simulink library "OFDM_Rx"  (R2020a)
settings: Solver=VariableStepAuto  StartTime=0.0  StopTime=10.0  RelTol=1e-3
undefined symbols (not defined in the file): fs, LTSfreq, pilot, read_addr_rx, sc_index
libraries: simulink x36, hdlsllib x24, dsphdlmathfun x3, dsphdlxfrm x1, dsphdlsigops x1
(part 2 of 3)

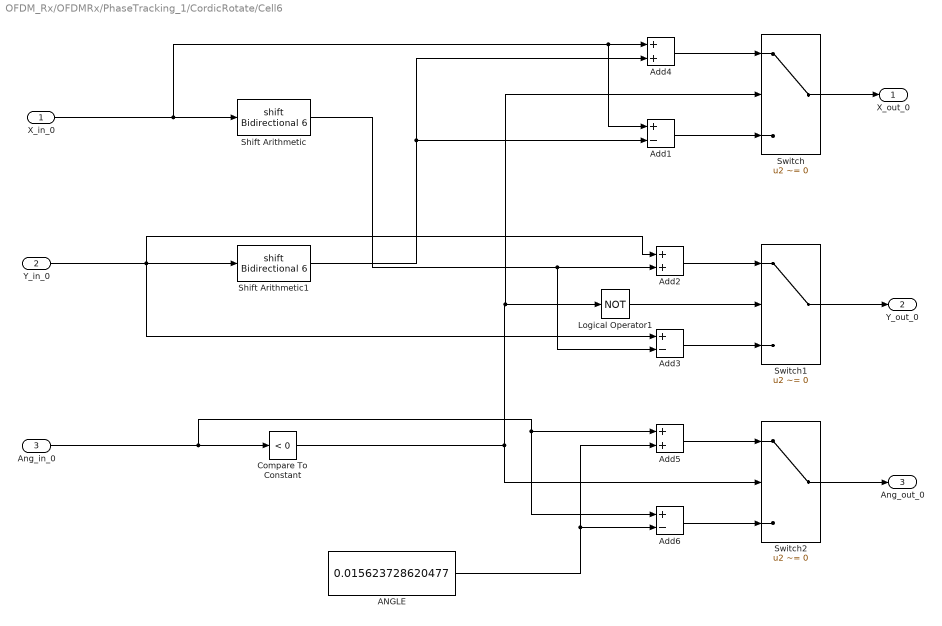
== system OFDM_Rx/OFDMRx/PhaseTracking_1/CordicRotate/Cell6 ==
  X_in_0 : Inport
  Y_in_0 : Inport  Port=2
  Ang_in_0 : Inport  Port=3
  ANGLE : Constant  Value=0.015623728620477  VectorParams1D=off  OutDataTypeStr=fixdt(1,23,20)  SampleTime=1/fs
  Add1 : Sum  Inputs=+-  OutDataTypeStr=fixdt(1,21,15)
  Add2 : Sum  OutDataTypeStr=fixdt(1,21,15)
  Add3 : Sum  Inputs=+-  OutDataTypeStr=fixdt(1,21,15)
  Add4 : Sum  OutDataTypeStr=fixdt(1,21,15)
  Add5 : Sum  OutDataTypeStr=fixdt(1,23,20)
  Add6 : Sum  Inputs=+-  OutDataTypeStr=fixdt(1,23,20)
  Compare To Constant : simulink/Logic and Bit Operations/Compare To Constant  relop=<  const=0  OutDataTypeStr=boolean
  Logical Operator1 : Logic  Operator=NOT  IconShape=distinctive  AllPortsSameDT=off  OutDataTypeStr=boolean
  Shift Arithmetic : ArithShift  BitShiftNumber=6
  Shift Arithmetic1 : ArithShift  BitShiftNumber=6
  Switch : Switch  Criteria=u2 ~= 0
  Switch1 : Switch  Criteria=u2 ~= 0
  Switch2 : Switch  Criteria=u2 ~= 0
  X_out_0 : Outport  VectorParamsAs1DForOutWhenUnconnected=off
  Y_out_0 : Outport  Port=2  VectorParamsAs1DForOutWhenUnconnected=off
  Ang_out_0 : Outport  Port=3  VectorParamsAs1DForOutWhenUnconnected=off
  wires:
  Add4/1 -> Switch/1
  Add1/1 -> Switch/3
  Add3/1 -> Switch1/3
  Add2/1 -> Switch1/1
  Switch/1 -> X_out_0/1
  Switch1/1 -> Y_out_0/1
  Add6/1 -> Switch2/3
  Add5/1 -> Switch2/1
  Switch2/1 -> Ang_out_0/1
  X_in_0/1 -> Shift Arithmetic/1, Add1/1, Add4/1
  Y_in_0/1 -> Shift Arithmetic1/1, Add3/1, Add2/1
  Ang_in_0/1 -> Add6/1, Add5/1, Compare To Constant/1
  Compare To Constant/1 -> Logical Operator1/1, Switch/2, Switch2/2
  Shift Arithmetic1/1 -> Add1/2, Add4/2
  Shift Arithmetic/1 -> Add3/2, Add2/2
  Logical Operator1/1 -> Switch1/2
  ANGLE/1 -> Add6/2, Add5/2

== system OFDM_Rx/OFDMRx/PhaseTracking_1/CordicRotate/Cell7 ==
  X_in_0 : Inport
  Y_in_0 : Inport  Port=2
  Ang_in_0 : Inport  Port=3
  ANGLE : Constant  Value=0.007812341060101  VectorParams1D=off  OutDataTypeStr=fixdt(1,23,20)  SampleTime=1/fs
  Add1 : Sum  Inputs=+-  OutDataTypeStr=fixdt(1,21,15)
  Add2 : Sum  OutDataTypeStr=fixdt(1,21,15)
  Add3 : Sum  Inputs=+-  OutDataTypeStr=fixdt(1,21,15)
  Add4 : Sum  OutDataTypeStr=fixdt(1,21,15)
  Add5 : Sum  OutDataTypeStr=fixdt(1,23,20)
  Add6 : Sum  Inputs=+-  OutDataTypeStr=fixdt(1,23,20)
  Compare To Constant : simulink/Logic and Bit Operations/Compare To Constant  relop=<  const=0  OutDataTypeStr=boolean
  Logical Operator1 : Logic  Operator=NOT  IconShape=distinctive  AllPortsSameDT=off  OutDataTypeStr=boolean
  Shift Arithmetic : ArithShift  BitShiftNumber=7
  Shift Arithmetic1 : ArithShift  BitShiftNumber=7
  Switch : Switch  Criteria=u2 ~= 0
  Switch1 : Switch  Criteria=u2 ~= 0
  Switch2 : Switch  Criteria=u2 ~= 0
  X_out_0 : Outport  VectorParamsAs1DForOutWhenUnconnected=off
  Y_out_0 : Outport  Port=2  VectorParamsAs1DForOutWhenUnconnected=off
  Ang_out_0 : Outport  Port=3  VectorParamsAs1DForOutWhenUnconnected=off
  wires:
  ANGLE/1 -> Add5/2, Add6/2
  Logical Operator1/1 -> Switch1/2
  Shift Arithmetic/1 -> Add2/2, Add3/2
  Shift Arithmetic1/1 -> Add4/2, Add1/2
  Compare To Constant/1 -> Switch2/2, Switch/2, Logical Operator1/1
  Ang_in_0/1 -> Compare To Constant/1, Add5/1, Add6/1
  Y_in_0/1 -> Add2/1, Add3/1, Shift Arithmetic1/1
  X_in_0/1 -> Add4/1, Add1/1, Shift Arithmetic/1
  Switch2/1 -> Ang_out_0/1
  Add5/1 -> Switch2/1
  Add6/1 -> Switch2/3
  Switch1/1 -> Y_out_0/1
  Switch/1 -> X_out_0/1
  Add2/1 -> Switch1/1
  Add3/1 -> Switch1/3
  Add1/1 -> Switch/3
  Add4/1 -> Switch/1

== system OFDM_Rx/OFDMRx/PhaseTracking_1/CordicRotate/Cell8 ==
  X_in_0 : Inport
  Y_in_0 : Inport  Port=2
  Ang_in_0 : Inport  Port=3
  ANGLE : Constant  Value=0.003906230131967  VectorParams1D=off  OutDataTypeStr=fixdt(1,23,20)  SampleTime=1/fs
  Add1 : Sum  Inputs=+-  OutDataTypeStr=fixdt(1,21,15)
  Add2 : Sum  OutDataTypeStr=fixdt(1,21,15)
  Add3 : Sum  Inputs=+-  OutDataTypeStr=fixdt(1,21,15)
  Add4 : Sum  OutDataTypeStr=fixdt(1,21,15)
  Add5 : Sum  OutDataTypeStr=fixdt(1,23,20)
  Add6 : Sum  Inputs=+-  OutDataTypeStr=fixdt(1,23,20)
  Compare To Constant : simulink/Logic and Bit Operations/Compare To Constant  relop=<  const=0  OutDataTypeStr=boolean
  Logical Operator1 : Logic  Operator=NOT  IconShape=distinctive  AllPortsSameDT=off  OutDataTypeStr=boolean
  Shift Arithmetic : ArithShift  BitShiftNumber=8
  Shift Arithmetic1 : ArithShift  BitShiftNumber=8
  Switch : Switch  Criteria=u2 ~= 0
  Switch1 : Switch  Criteria=u2 ~= 0
  Switch2 : Switch  Criteria=u2 ~= 0
  X_out_0 : Outport  VectorParamsAs1DForOutWhenUnconnected=off
  Y_out_0 : Outport  Port=2  VectorParamsAs1DForOutWhenUnconnected=off
  Ang_out_0 : Outport  Port=3  VectorParamsAs1DForOutWhenUnconnected=off
  wires:
  Add4/1 -> Switch/1
  Add1/1 -> Switch/3
  Add3/1 -> Switch1/3
  Add2/1 -> Switch1/1
  Switch/1 -> X_out_0/1
  Switch1/1 -> Y_out_0/1
  Add6/1 -> Switch2/3
  Add5/1 -> Switch2/1
  Switch2/1 -> Ang_out_0/1
  X_in_0/1 -> Shift Arithmetic/1, Add1/1, Add4/1
  Y_in_0/1 -> Shift Arithmetic1/1, Add3/1, Add2/1
  Ang_in_0/1 -> Add6/1, Add5/1, Compare To Constant/1
  Compare To Constant/1 -> Logical Operator1/1, Switch/2, Switch2/2
  Shift Arithmetic1/1 -> Add1/2, Add4/2
  Shift Arithmetic/1 -> Add3/2, Add2/2
  Logical Operator1/1 -> Switch1/2
  ANGLE/1 -> Add6/2, Add5/2

== system OFDM_Rx/OFDMRx/PhaseTracking_1/CordicRotate/Cell9 ==
  X_in_0 : Inport
  Y_in_0 : Inport  Port=2
  Ang_in_0 : Inport  Port=3
  ANGLE : Constant  Value=0.001953122516479  VectorParams1D=off  OutDataTypeStr=fixdt(1,23,20)  SampleTime=1/fs
  Add1 : Sum  Inputs=+-  OutDataTypeStr=fixdt(1,21,15)
  Add2 : Sum  OutDataTypeStr=fixdt(1,21,15)
  Add3 : Sum  Inputs=+-  OutDataTypeStr=fixdt(1,21,15)
  Add4 : Sum  OutDataTypeStr=fixdt(1,21,15)
  Add5 : Sum  OutDataTypeStr=fixdt(1,23,20)
  Add6 : Sum  Inputs=+-  OutDataTypeStr=fixdt(1,23,20)
  Compare To Constant : simulink/Logic and Bit Operations/Compare To Constant  relop=<  const=0  OutDataTypeStr=boolean
  Logical Operator1 : Logic  Operator=NOT  IconShape=distinctive  AllPortsSameDT=off  OutDataTypeStr=boolean
  Shift Arithmetic : ArithShift  BitShiftNumber=9
  Shift Arithmetic1 : ArithShift  BitShiftNumber=9
  Switch : Switch  Criteria=u2 ~= 0
  Switch1 : Switch  Criteria=u2 ~= 0
  Switch2 : Switch  Criteria=u2 ~= 0
  X_out_0 : Outport  VectorParamsAs1DForOutWhenUnconnected=off
  Y_out_0 : Outport  Port=2  VectorParamsAs1DForOutWhenUnconnected=off
  Ang_out_0 : Outport  Port=3  VectorParamsAs1DForOutWhenUnconnected=off
  wires:
  ANGLE/1 -> Add5/2, Add6/2
  Logical Operator1/1 -> Switch1/2
  Shift Arithmetic/1 -> Add2/2, Add3/2
  Shift Arithmetic1/1 -> Add4/2, Add1/2
  Compare To Constant/1 -> Switch2/2, Switch/2, Logical Operator1/1
  Ang_in_0/1 -> Compare To Constant/1, Add5/1, Add6/1
  Y_in_0/1 -> Add2/1, Add3/1, Shift Arithmetic1/1
  X_in_0/1 -> Add4/1, Add1/1, Shift Arithmetic/1
  Switch2/1 -> Ang_out_0/1
  Add5/1 -> Switch2/1
  Add6/1 -> Switch2/3
  Switch1/1 -> Y_out_0/1
  Switch/1 -> X_out_0/1
  Add2/1 -> Switch1/1
  Add3/1 -> Switch1/3
  Add1/1 -> Switch/3
  Add4/1 -> Switch/1

== system OFDM_Rx/OFDMRx/PhaseTracking_1/CordicRotate/GAIN_CORR ==
  XIN : Inport
  Constant : Constant  Value=0.607253321089875  OutDataTypeStr=fixdt(1,18,17)  SampleTime=1/fs
  Data Type Conversion : DataTypeConversion  OutDataTypeStr=fixdt(1,18,15)
  Product : Product
  XOUT : Outport  VectorParamsAs1DForOutWhenUnconnected=off
  wires:
  Data Type Conversion/1 -> XOUT/1
  XIN/1 -> Product/2
  Constant/1 -> Product/1
  Product/1 -> Data Type Conversion/1

== system OFDM_Rx/OFDMRx/PhaseTracking_1/CordicRotate/GAIN_CORR1 ==
  YIN : Inport
  Constant : Constant  Value=0.607253321089875  OutDataTypeStr=fixdt(1,18,17)  SampleTime=1/fs
  Data Type Conversion : DataTypeConversion  OutDataTypeStr=fixdt(1,18,15)
  Product : Product
  YOUT : Outport  VectorParamsAs1DForOutWhenUnconnected=off
  wires:
  Data Type Conversion/1 -> YOUT/1
  Product/1 -> Data Type Conversion/1
  Constant/1 -> Product/1
  YIN/1 -> Product/2

== system OFDM_Rx/OFDMRx/PhaseTracking_1/CordicRotate/QCORR ==
  X_in : Inport
  Y_in : Inport  Port=2
  Ctrl_in : Inport  Port=3
  QUAD_MAP1 : MATLAB Function  TreatAsAtomicUnit=on
  X_out : Outport  VectorParamsAs1DForOutWhenUnconnected=off
  Y_out : Outport  Port=2  VectorParamsAs1DForOutWhenUnconnected=off
  wires:
  Ctrl_in/1 -> QUAD_MAP1/3(ctrl)
  Y_in/1 -> QUAD_MAP1/2(yin)
  X_in/1 -> QUAD_MAP1/1(xin)
  QUAD_MAP1/1(xout) -> X_out/1
  QUAD_MAP1/2(yout) -> Y_out/1

== system OFDM_Rx/OFDMRx/PhaseTracking_1/CordicRotate/QUAD_MAP ==
  Xin : Inport
  Yin : Inport  Port=2
  ANG_IN : Inport  Port=3
  QUAD_DETERM1 : MATLAB Function  TreatAsAtomicUnit=on
  Xout : Outport  VectorParamsAs1DForOutWhenUnconnected=off
  Yout : Outport  Port=2  VectorParamsAs1DForOutWhenUnconnected=off
  ANG_OUT : Outport  Port=3  VectorParamsAs1DForOutWhenUnconnected=off
  QUAD_CTRL_OUT : Outport  Port=4  VectorParamsAs1DForOutWhenUnconnected=off
  wires:
  ANG_IN/1 -> QUAD_DETERM1/1(ang_in)
  QUAD_DETERM1/1(ang_out) -> ANG_OUT/1
  Xin/1 -> Xout/1
  Yin/1 -> Yout/1
  QUAD_DETERM1/2(QUAD) -> QUAD_CTRL_OUT/1

== system OFDM_Rx/OFDMRx/PhaseTracking_1/DataArrange/READ_CTRL ==
  In1 : Inport
  In2 : Inport  Port=2
  Constant : Constant  Value=0  OutDataTypeStr=fixdt(0,7,0)  SampleTime=1/fs
  Switch : Switch  Criteria=u2 ~= 0
  Out1 : Outport  VectorParamsAs1DForOutWhenUnconnected=off
  wires:
  Switch/1 -> Out1/1
  In1/1 -> Switch/1
  In2/1 -> Switch/2
  Constant/1 -> Switch/3

== system OFDM_Rx/OFDMRx/PhaseTracking_1/DataArrange/dataValidGen ==
  enb : Inport
  AND : Logic  IconShape=distinctive  AllPortsSameDT=off  OutDataTypeStr=boolean
  Compare To Constant : simulink/Logic and Bit Operations/Compare To Constant  relop=>  const=11  OutDataTypeStr=boolean
  HDL Counter2 : hdlsllib/Sources/HDL Counter  CountType=Count limited  CountInit=0  CountStep=1  CountMax=63  CountFromType=Initial value  CountFrom=0  CountResetPort=on  CountLoadPort=off  CountEnbPort=on  CountDirPort=off  CountDataType=Unsigned  CountWordLen=8  CountFracLen=0  CountSampTime=1
  NOT : Logic  Operator=NOT  IconShape=distinctive  AllPortsSameDT=off  OutDataTypeStr=boolean
  dataValidOut : Outport
  wires:
  Compare To Constant/1 -> AND/1
  AND/1 -> dataValidOut/1
  enb/1 -> HDL Counter2/2, NOT/1, AND/2
  HDL Counter2/1 -> Compare To Constant/1
  NOT/1 -> HDL Counter2/1

== system OFDM_Rx/OFDMRx/PhaseTracking_1/GradientEstimate /Gradient ==
  note: Estimate gardient of phase slope using . The no. of
      | gradient estimates is 3 since there are 4 pilots.
  diffIn : Inport
  Add : Sum  Inputs=+-  OutDataTypeStr=fixdt(1,28,20)
  Delay1 : Delay  DelayLength=1
  Delay2 : Delay  DelayLength=1
  Delay3 : Delay  DelayLength=1
  Gain : Gain  Gain=1/14  OutDataTypeStr=fixdt(1,23,20)
  diffOut : Outport
  wires:
  Gain/1 -> Delay3/1
  diffIn/1 -> Delay2/1
  Add/1 -> Gain/1
  Delay1/1 -> Add/1
  Delay2/1 -> Add/2, Delay1/1
  Delay3/1 -> diffOut/1

== system OFDM_Rx/OFDMRx/PhaseTracking_1/GradientEstimate /MoveAvg ==
  note: Average the gradient estimates to reduce
      | effects of noise as much as possible.
  mvAvgIn : Inport
  Add : Sum  Inputs=-+  AccumDataTypeStr=fixdt(1,25,20)
  Add1 : Sum  AccumDataTypeStr=fixdt(1,25,20)
  Delay1 : Delay  DelayLength=3
  Delay2 : Delay  DelayLength=1
  Gain : Gain  Gain=1/3  OutDataTypeStr=fixdt(1,23,20)
  mvAvgOut : Outport  VectorParamsAs1DForOutWhenUnconnected=off
  wires:
  Delay2/1 -> Gain/1, Add1/1
  mvAvgIn/1 -> Delay1/1, Add/2
  Delay1/1 -> Add/1
  Add/1 -> Add1/2
  Add1/1 -> Delay2/1
  Gain/1 -> mvAvgOut/1

== system OFDM_Rx/OFDMRx/PhaseTracking_1/GradientEstimate /PilotEq ==
  In1 : Inport
  In2 : Inport  Port=2
  Delay2 : Delay  DelayLength=1
  Delay3 : Delay  DelayLength=1
  Delay5 : Delay  DelayLength=1
  Product : Product  OutDataTypeStr=fixdt(1,18,15)
  Out1 : Outport
  wires:
  Product/1 -> Delay5/1
  In2/1 -> Delay3/1
  In1/1 -> Delay2/1
  Delay3/1 -> Product/2
  Delay5/1 -> Out1/1
  Delay2/1 -> Product/1

== system OFDM_Rx/OFDMRx/PhaseTracking_1/PilotCtrlGen/CtrlSigGen ==
  valid : Inport
  sampleCount : Inport  Port=2
  Compare To Constant1 : simulink/Logic and Bit Operations/Compare To Constant  relop===  const=3  OutDataTypeStr=boolean
  Logical Operator5 : Logic  IconShape=distinctive  AllPortsSameDT=off  OutDataTypeStr=boolean
  dataValid : Outport
  pilotEnd : Outport  Port=2
  wires:
  sampleCount/1 -> Compare To Constant1/1
  valid/1 -> dataValid/1, Logical Operator5/1
  Compare To Constant1/1 -> Logical Operator5/2
  Logical Operator5/1 -> pilotEnd/1

== system OFDM_Rx/OFDMRx/PhaseTracking_1/PilotCtrlGen/SampleCounter ==
  Valid_In : Inport
  Delay : Delay  DelayLength=1
  Logical Operator : Logic  Operator=NOT  IconShape=distinctive  AllPortsSameDT=off  OutDataTypeStr=boolean
  SAMPLE_COUNTER : hdlsllib/Sources/HDL Counter  CountType=Count limited  CountInit=0  CountStep=1  CountMax=51  CountFromType=Initial value  CountFrom=0  CountResetPort=on  CountLoadPort=off  CountEnbPort=on  CountDirPort=off  CountDataType=Unsigned  CountWordLen=6  CountFracLen=0  CountSampTime=1
  Sample_Cnt : Outport  VectorParamsAs1DForOutWhenUnconnected=off
  wires:
  Delay/1 -> Sample_Cnt/1
  Logical Operator/1 -> SAMPLE_COUNTER/1
  Valid_In/1 -> SAMPLE_COUNTER/2, Logical Operator/1
  SAMPLE_COUNTER/1 -> Delay/1

== system OFDM_Rx/OFDMRx/PhaseTracking_1/PilotCtrlGen/SymbolCounter ==
  ValidIn : Inport
  Delay : Delay  DelayLength=1
  HDL Counter : hdlsllib/Sources/HDL Counter  CountType=Count limited  CountInit=0  CountStep=1  CountMax=126  CountFromType=Initial value  CountFrom=0  CountResetPort=off  CountLoadPort=off  CountEnbPort=on  CountDirPort=off  CountDataType=Unsigned  CountWordLen=7  CountFracLen=0  CountSampTime=1
  Relational Operator : RelationalOperator  Operator=<  OutDataTypeStr=boolean  RndMeth=Nearest
  Symbl_cnt : Outport  VectorParamsAs1DForOutWhenUnconnected=off
  wires:
  Relational Operator/1 -> HDL Counter/1
  HDL Counter/1 -> Symbl_cnt/1
  Delay/1 -> Relational Operator/2
  ValidIn/1 -> Delay/1, Relational Operator/1

== system OFDM_Rx/OFDMRx/PhaseTracking_1/PilotCtrlGen/pilotGen ==
  symbCount : Inport
  sampleCount : Inport  Port=2
  valid : Inport  Port=3
  Compare To Constant : simulink/Logic and Bit Operations/Compare To Constant  relop=>  const=0  OutDataTypeStr=boolean
  Compare To Constant2 : simulink/Logic and Bit Operations/Compare To Constant  relop=>=  const=0  OutDataTypeStr=boolean
  Compare To Constant3 : simulink/Logic and Bit Operations/Compare To Constant  relop=<  const=4  OutDataTypeStr=boolean
  Constant : Constant  Value=0  OutDataTypeStr=fixdt(1,2,0)  SampleTime=1/fs
  HDL Counter1 : hdlsllib/Sources/HDL Counter  CountType=Count limited  CountInit=0  CountStep=1  CountMax=3  CountFromType=Initial value  CountFrom=0  CountResetPort=off  CountLoadPort=off  CountEnbPort=on  CountDirPort=off  CountDataType=Unsigned  CountWordLen=2  CountFracLen=0  CountSampTime=1
  Logical Operator1 : Logic  IconShape=distinctive  AllPortsSameDT=off  OutDataTypeStr=boolean
  Logical Operator3 : Logic  IconShape=distinctive  AllPortsSameDT=off  OutDataTypeStr=boolean
  PilotValue_LUT1 : Lookup_n-D  NumberOfTableDimensions=1  LookupTableObject=''  BreakpointsForDimension1=[0:3]  BreakpointsForDimension1FirstPoint=10  BreakpointsForDimension2FirstPoint=10  BreakpointsForDimension1Spacing=12  BreakpointsForDimension2Spacing=12  IndexSearchMethod=Evenly spaced points  Table=[1 1 1 -1]  TableDataTypeStr=fixdt(1,2,0)  InterpMethod=Flat  DiagnosticForOutOfRangeInput=Error  InternalRulePriority=Speed  OutDataTypeStr=fixdt(1,2,0)  RndMeth=Simplest  InputSameDT=on
  Polarity_LUT1 : Lookup_n-D  NumberOfTableDimensions=1  LookupTableObject=''  BreakpointsForDimension1=[0:126]  BreakpointsForDimension1FirstPoint=10  BreakpointsForDimension2FirstPoint=10  BreakpointsForDimension1Spacing=12  BreakpointsForDimension2Spacing=12  IndexSearchMethod=Evenly spaced points  Table=pilot  TableDataTypeStr=fixdt(1,2,0)  InterpMethod=Flat  DiagnosticForOutOfRangeInput=Error  InternalRulePriority=Speed  OutDataTypeStr=fixdt(1,2,0)  RndMeth=Simplest  InputSameDT=on
  Switch : Switch  Criteria=u2 ~= 0
  Switch1 : Switch  Criteria=u2 ~= 0
  ToComplex1 : Subsystem
  Unary Minus : UnaryMinus
  pilOut : Outport
  wires:
  Logical Operator3/1 -> HDL Counter1/1, Switch1/2
  valid/1 -> Logical Operator3/1
  Compare To Constant3/1 -> Logical Operator1/2
  Compare To Constant2/1 -> Logical Operator1/1
  Logical Operator1/1 -> Logical Operator3/2
  sampleCount/1 -> Compare To Constant3/1, Compare To Constant2/1
  symbCount/1 -> Polarity_LUT1/1
  Constant/1 -> Switch1/3
  Switch1/1 -> Switch/1, Unary Minus/1
  ToComplex1/1(Out1) -> pilOut/1
  Compare To Constant/1 -> Switch/2
  Unary Minus/1 -> Switch/3
  Switch/1 -> ToComplex1/1(In1)
  PilotValue_LUT1/1 -> Switch1/1
  Polarity_LUT1/1 -> Compare To Constant/1
  HDL Counter1/1 -> PilotValue_LUT1/1

== system OFDM_Rx/OFDMRx/PhaseTracking_2/CordicRotate/Cell0 ==
  X_in_0 : Inport
  Y_in_0 : Inport  Port=2
  Ang_in_0 : Inport  Port=3
  ANGLE : Constant  Value=0.785398163397448  VectorParams1D=off  OutDataTypeStr=fixdt(1,23,20)  SampleTime=1/fs
  Add1 : Sum  Inputs=+-  OutDataTypeStr=fixdt(1,21,15)
  Add2 : Sum  OutDataTypeStr=fixdt(1,21,15)
  Add3 : Sum  Inputs=+-  OutDataTypeStr=fixdt(1,21,15)
  Add4 : Sum  OutDataTypeStr=fixdt(1,21,15)
  Add5 : Sum  OutDataTypeStr=fixdt(1,23,20)
  Add6 : Sum  Inputs=+-  OutDataTypeStr=fixdt(1,23,20)
  Compare To Constant : simulink/Logic and Bit Operations/Compare To Constant  relop=<  const=0  OutDataTypeStr=boolean
  Logical Operator1 : Logic  Operator=NOT  IconShape=distinctive  AllPortsSameDT=off  OutDataTypeStr=boolean
  Shift Arithmetic : ArithShift
  Shift Arithmetic1 : ArithShift
  Switch : Switch  Criteria=u2 ~= 0
  Switch1 : Switch  Criteria=u2 ~= 0
  Switch2 : Switch  Criteria=u2 ~= 0
  X_out_0 : Outport  VectorParamsAs1DForOutWhenUnconnected=off
  Y_out_0 : Outport  Port=2  VectorParamsAs1DForOutWhenUnconnected=off
  Ang_out_0 : Outport  Port=3  VectorParamsAs1DForOutWhenUnconnected=off
  wires:
  Add4/1 -> Switch/1
  Add1/1 -> Switch/3
  Add3/1 -> Switch1/3
  Add2/1 -> Switch1/1
  Switch/1 -> X_out_0/1
  Switch1/1 -> Y_out_0/1
  Add6/1 -> Switch2/3
  Add5/1 -> Switch2/1
  Switch2/1 -> Ang_out_0/1
  X_in_0/1 -> Shift Arithmetic/1, Add1/1, Add4/1
  Y_in_0/1 -> Shift Arithmetic1/1, Add3/1, Add2/1
  Ang_in_0/1 -> Add6/1, Add5/1, Compare To Constant/1
  Compare To Constant/1 -> Logical Operator1/1, Switch/2, Switch2/2
  Shift Arithmetic1/1 -> Add1/2, Add4/2
  Shift Arithmetic/1 -> Add3/2, Add2/2
  Logical Operator1/1 -> Switch1/2
  ANGLE/1 -> Add6/2, Add5/2

== system OFDM_Rx/OFDMRx/PhaseTracking_2/CordicRotate/Cell1 ==
  X_in_0 : Inport
  Y_in_0 : Inport  Port=2
  Ang_in_0 : Inport  Port=3
  ANGLE : Constant  Value=0.463647609000806  VectorParams1D=off  OutDataTypeStr=fixdt(1,23,20)  SampleTime=1/fs
  Add1 : Sum  Inputs=+-  OutDataTypeStr=fixdt(1,21,15)
  Add2 : Sum  OutDataTypeStr=fixdt(1,21,15)
  Add3 : Sum  Inputs=+-  OutDataTypeStr=fixdt(1,21,15)
  Add4 : Sum  OutDataTypeStr=fixdt(1,21,15)
  Add5 : Sum  OutDataTypeStr=fixdt(1,23,20)
  Add6 : Sum  Inputs=+-  OutDataTypeStr=fixdt(1,23,20)
  Compare To Constant : simulink/Logic and Bit Operations/Compare To Constant  relop=<  const=0  OutDataTypeStr=boolean
  Logical Operator1 : Logic  Operator=NOT  IconShape=distinctive  AllPortsSameDT=off  OutDataTypeStr=boolean
  Shift Arithmetic : ArithShift  BitShiftNumber=1
  Shift Arithmetic1 : ArithShift  BitShiftNumber=1
  Switch : Switch  Criteria=u2 ~= 0
  Switch1 : Switch  Criteria=u2 ~= 0
  Switch2 : Switch  Criteria=u2 ~= 0
  X_out_0 : Outport  VectorParamsAs1DForOutWhenUnconnected=off
  Y_out_0 : Outport  Port=2  VectorParamsAs1DForOutWhenUnconnected=off
  Ang_out_0 : Outport  Port=3  VectorParamsAs1DForOutWhenUnconnected=off
  wires:
  ANGLE/1 -> Add5/2, Add6/2
  Logical Operator1/1 -> Switch1/2
  Shift Arithmetic/1 -> Add2/2, Add3/2
  Shift Arithmetic1/1 -> Add4/2, Add1/2
  Compare To Constant/1 -> Switch2/2, Switch/2, Logical Operator1/1
  Ang_in_0/1 -> Compare To Constant/1, Add5/1, Add6/1
  Y_in_0/1 -> Add2/1, Add3/1, Shift Arithmetic1/1
  X_in_0/1 -> Add4/1, Add1/1, Shift Arithmetic/1
  Switch2/1 -> Ang_out_0/1
  Add5/1 -> Switch2/1
  Add6/1 -> Switch2/3
  Switch1/1 -> Y_out_0/1
  Switch/1 -> X_out_0/1
  Add2/1 -> Switch1/1
  Add3/1 -> Switch1/3
  Add1/1 -> Switch/3
  Add4/1 -> Switch/1

== system OFDM_Rx/OFDMRx/PhaseTracking_2/CordicRotate/Cell2 ==
  X_in_0 : Inport
  Y_in_0 : Inport  Port=2
  Ang_in_0 : Inport  Port=3
  ANGLE : Constant  Value=0.244978663126864  VectorParams1D=off  OutDataTypeStr=fixdt(1,23,20)  SampleTime=1/fs
  Add1 : Sum  Inputs=+-  OutDataTypeStr=fixdt(1,21,15)
  Add2 : Sum  OutDataTypeStr=fixdt(1,21,15)
  Add3 : Sum  Inputs=+-  OutDataTypeStr=fixdt(1,21,15)
  Add4 : Sum  OutDataTypeStr=fixdt(1,21,15)
  Add5 : Sum  OutDataTypeStr=fixdt(1,23,20)
  Add6 : Sum  Inputs=+-  OutDataTypeStr=fixdt(1,23,20)
  Compare To Constant : simulink/Logic and Bit Operations/Compare To Constant  relop=<  const=0  OutDataTypeStr=boolean
  Logical Operator1 : Logic  Operator=NOT  IconShape=distinctive  AllPortsSameDT=off  OutDataTypeStr=boolean
  Shift Arithmetic : ArithShift  BitShiftNumber=2
  Shift Arithmetic1 : ArithShift  BitShiftNumber=2
  Switch : Switch  Criteria=u2 ~= 0
  Switch1 : Switch  Criteria=u2 ~= 0
  Switch2 : Switch  Criteria=u2 ~= 0
  X_out_0 : Outport  VectorParamsAs1DForOutWhenUnconnected=off
  Y_out_0 : Outport  Port=2  VectorParamsAs1DForOutWhenUnconnected=off
  Ang_out_0 : Outport  Port=3  VectorParamsAs1DForOutWhenUnconnected=off
  wires:
  Add4/1 -> Switch/1
  Add1/1 -> Switch/3
  Add3/1 -> Switch1/3
  Add2/1 -> Switch1/1
  Switch/1 -> X_out_0/1
  Switch1/1 -> Y_out_0/1
  Add6/1 -> Switch2/3
  Add5/1 -> Switch2/1
  Switch2/1 -> Ang_out_0/1
  X_in_0/1 -> Shift Arithmetic/1, Add1/1, Add4/1
  Y_in_0/1 -> Shift Arithmetic1/1, Add3/1, Add2/1
  Ang_in_0/1 -> Add6/1, Add5/1, Compare To Constant/1
  Compare To Constant/1 -> Logical Operator1/1, Switch/2, Switch2/2
  Shift Arithmetic1/1 -> Add1/2, Add4/2
  Shift Arithmetic/1 -> Add3/2, Add2/2
  Logical Operator1/1 -> Switch1/2
  ANGLE/1 -> Add6/2, Add5/2

== system OFDM_Rx/OFDMRx/PhaseTracking_2/CordicRotate/Cell3 ==
  X_in_0 : Inport
  Y_in_0 : Inport  Port=2
  Ang_in_0 : Inport  Port=3
  ANGLE : Constant  Value=0.124354994546761  VectorParams1D=off  OutDataTypeStr=fixdt(1,23,20)  SampleTime=1/fs
  Add1 : Sum  Inputs=+-  OutDataTypeStr=fixdt(1,21,15)
  Add2 : Sum  OutDataTypeStr=fixdt(1,21,15)
  Add3 : Sum  Inputs=+-  OutDataTypeStr=fixdt(1,21,15)
  Add4 : Sum  OutDataTypeStr=fixdt(1,21,15)
  Add5 : Sum  OutDataTypeStr=fixdt(1,23,20)
  Add6 : Sum  Inputs=+-  OutDataTypeStr=fixdt(1,23,20)
  Compare To Constant : simulink/Logic and Bit Operations/Compare To Constant  relop=<  const=0  OutDataTypeStr=boolean
  Logical Operator1 : Logic  Operator=NOT  IconShape=distinctive  AllPortsSameDT=off  OutDataTypeStr=boolean
  Shift Arithmetic : ArithShift  BitShiftNumber=3
  Shift Arithmetic1 : ArithShift  BitShiftNumber=3
  Switch : Switch  Criteria=u2 ~= 0
  Switch1 : Switch  Criteria=u2 ~= 0
  Switch2 : Switch  Criteria=u2 ~= 0
  X_out_0 : Outport  VectorParamsAs1DForOutWhenUnconnected=off
  Y_out_0 : Outport  Port=2  VectorParamsAs1DForOutWhenUnconnected=off
  Ang_out_0 : Outport  Port=3  VectorParamsAs1DForOutWhenUnconnected=off
  wires:
  ANGLE/1 -> Add5/2, Add6/2
  Logical Operator1/1 -> Switch1/2
  Shift Arithmetic/1 -> Add2/2, Add3/2
  Shift Arithmetic1/1 -> Add4/2, Add1/2
  Compare To Constant/1 -> Switch2/2, Switch/2, Logical Operator1/1
  Ang_in_0/1 -> Compare To Constant/1, Add5/1, Add6/1
  Y_in_0/1 -> Add2/1, Add3/1, Shift Arithmetic1/1
  X_in_0/1 -> Add4/1, Add1/1, Shift Arithmetic/1
  Switch2/1 -> Ang_out_0/1
  Add5/1 -> Switch2/1
  Add6/1 -> Switch2/3
  Switch1/1 -> Y_out_0/1
  Switch/1 -> X_out_0/1
  Add2/1 -> Switch1/1
  Add3/1 -> Switch1/3
  Add1/1 -> Switch/3
  Add4/1 -> Switch/1

== system OFDM_Rx/OFDMRx/PhaseTracking_2/CordicRotate/Cell4 ==
  X_in_0 : Inport
  Y_in_0 : Inport  Port=2
  Ang_in_0 : Inport  Port=3
  ANGLE : Constant  Value=0.062418809995957  VectorParams1D=off  OutDataTypeStr=fixdt(1,23,20)  SampleTime=1/fs
  Add1 : Sum  Inputs=+-  OutDataTypeStr=fixdt(1,21,15)
  Add2 : Sum  OutDataTypeStr=fixdt(1,21,15)
  Add3 : Sum  Inputs=+-  OutDataTypeStr=fixdt(1,21,15)
  Add4 : Sum  OutDataTypeStr=fixdt(1,21,15)
  Add5 : Sum  OutDataTypeStr=fixdt(1,23,20)
  Add6 : Sum  Inputs=+-  OutDataTypeStr=fixdt(1,23,20)
  Compare To Constant : simulink/Logic and Bit Operations/Compare To Constant  relop=<  const=0  OutDataTypeStr=boolean
  Logical Operator1 : Logic  Operator=NOT  IconShape=distinctive  AllPortsSameDT=off  OutDataTypeStr=boolean
  Shift Arithmetic : ArithShift  BitShiftNumber=4
  Shift Arithmetic1 : ArithShift  BitShiftNumber=4
  Switch : Switch  Criteria=u2 ~= 0
  Switch1 : Switch  Criteria=u2 ~= 0
  Switch2 : Switch  Criteria=u2 ~= 0
  X_out_0 : Outport  VectorParamsAs1DForOutWhenUnconnected=off
  Y_out_0 : Outport  Port=2  VectorParamsAs1DForOutWhenUnconnected=off
  Ang_out_0 : Outport  Port=3  VectorParamsAs1DForOutWhenUnconnected=off
  wires:
  Add4/1 -> Switch/1
  Add1/1 -> Switch/3
  Add3/1 -> Switch1/3
  Add2/1 -> Switch1/1
  Switch/1 -> X_out_0/1
  Switch1/1 -> Y_out_0/1
  Add6/1 -> Switch2/3
  Add5/1 -> Switch2/1
  Switch2/1 -> Ang_out_0/1
  X_in_0/1 -> Shift Arithmetic/1, Add1/1, Add4/1
  Y_in_0/1 -> Shift Arithmetic1/1, Add3/1, Add2/1
  Ang_in_0/1 -> Add6/1, Add5/1, Compare To Constant/1
  Compare To Constant/1 -> Logical Operator1/1, Switch/2, Switch2/2
  Shift Arithmetic1/1 -> Add1/2, Add4/2
  Shift Arithmetic/1 -> Add3/2, Add2/2
  Logical Operator1/1 -> Switch1/2
  ANGLE/1 -> Add6/2, Add5/2

== system OFDM_Rx/OFDMRx/PhaseTracking_2/CordicRotate/Cell5 ==
  X_in_0 : Inport
  Y_in_0 : Inport  Port=2
  Ang_in_0 : Inport  Port=3
  ANGLE : Constant  Value=0.031239833430268  VectorParams1D=off  OutDataTypeStr=fixdt(1,23,20)  SampleTime=1/fs
  Add1 : Sum  Inputs=+-  OutDataTypeStr=fixdt(1,21,15)
  Add2 : Sum  OutDataTypeStr=fixdt(1,21,15)
  Add3 : Sum  Inputs=+-  OutDataTypeStr=fixdt(1,21,15)
  Add4 : Sum  OutDataTypeStr=fixdt(1,21,15)
  Add5 : Sum  OutDataTypeStr=fixdt(1,23,20)
  Add6 : Sum  Inputs=+-  OutDataTypeStr=fixdt(1,23,20)
  Compare To Constant : simulink/Logic and Bit Operations/Compare To Constant  relop=<  const=0  OutDataTypeStr=boolean
  Logical Operator1 : Logic  Operator=NOT  IconShape=distinctive  AllPortsSameDT=off  OutDataTypeStr=boolean
  Shift Arithmetic : ArithShift  BitShiftNumber=5
  Shift Arithmetic1 : ArithShift  BitShiftNumber=5
  Switch : Switch  Criteria=u2 ~= 0
  Switch1 : Switch  Criteria=u2 ~= 0
  Switch2 : Switch  Criteria=u2 ~= 0
  X_out_0 : Outport  VectorParamsAs1DForOutWhenUnconnected=off
  Y_out_0 : Outport  Port=2  VectorParamsAs1DForOutWhenUnconnected=off
  Ang_out_0 : Outport  Port=3  VectorParamsAs1DForOutWhenUnconnected=off
  wires:
  ANGLE/1 -> Add5/2, Add6/2
  Logical Operator1/1 -> Switch1/2
  Shift Arithmetic/1 -> Add2/2, Add3/2
  Shift Arithmetic1/1 -> Add4/2, Add1/2
  Compare To Constant/1 -> Switch2/2, Switch/2, Logical Operator1/1
  Ang_in_0/1 -> Compare To Constant/1, Add5/1, Add6/1
  Y_in_0/1 -> Add2/1, Add3/1, Shift Arithmetic1/1
  X_in_0/1 -> Add4/1, Add1/1, Shift Arithmetic/1
  Switch2/1 -> Ang_out_0/1
  Add5/1 -> Switch2/1
  Add6/1 -> Switch2/3
  Switch1/1 -> Y_out_0/1
  Switch/1 -> X_out_0/1
  Add2/1 -> Switch1/1
  Add3/1 -> Switch1/3
  Add1/1 -> Switch/3
  Add4/1 -> Switch/1

== system OFDM_Rx/OFDMRx/PhaseTracking_2/CordicRotate/Cell6 ==
  X_in_0 : Inport
  Y_in_0 : Inport  Port=2
  Ang_in_0 : Inport  Port=3
  ANGLE : Constant  Value=0.015623728620477  VectorParams1D=off  OutDataTypeStr=fixdt(1,23,20)  SampleTime=1/fs
  Add1 : Sum  Inputs=+-  OutDataTypeStr=fixdt(1,21,15)
  Add2 : Sum  OutDataTypeStr=fixdt(1,21,15)
  Add3 : Sum  Inputs=+-  OutDataTypeStr=fixdt(1,21,15)
  Add4 : Sum  OutDataTypeStr=fixdt(1,21,15)
  Add5 : Sum  OutDataTypeStr=fixdt(1,23,20)
  Add6 : Sum  Inputs=+-  OutDataTypeStr=fixdt(1,23,20)
  Compare To Constant : simulink/Logic and Bit Operations/Compare To Constant  relop=<  const=0  OutDataTypeStr=boolean
  Logical Operator1 : Logic  Operator=NOT  IconShape=distinctive  AllPortsSameDT=off  OutDataTypeStr=boolean
  Shift Arithmetic : ArithShift  BitShiftNumber=6
  Shift Arithmetic1 : ArithShift  BitShiftNumber=6
  Switch : Switch  Criteria=u2 ~= 0
  Switch1 : Switch  Criteria=u2 ~= 0
  Switch2 : Switch  Criteria=u2 ~= 0
  X_out_0 : Outport  VectorParamsAs1DForOutWhenUnconnected=off
  Y_out_0 : Outport  Port=2  VectorParamsAs1DForOutWhenUnconnected=off
  Ang_out_0 : Outport  Port=3  VectorParamsAs1DForOutWhenUnconnected=off
  wires:
  Add4/1 -> Switch/1
  Add1/1 -> Switch/3
  Add3/1 -> Switch1/3
  Add2/1 -> Switch1/1
  Switch/1 -> X_out_0/1
  Switch1/1 -> Y_out_0/1
  Add6/1 -> Switch2/3
  Add5/1 -> Switch2/1
  Switch2/1 -> Ang_out_0/1
  X_in_0/1 -> Shift Arithmetic/1, Add1/1, Add4/1
  Y_in_0/1 -> Shift Arithmetic1/1, Add3/1, Add2/1
  Ang_in_0/1 -> Add6/1, Add5/1, Compare To Constant/1
  Compare To Constant/1 -> Logical Operator1/1, Switch/2, Switch2/2
  Shift Arithmetic1/1 -> Add1/2, Add4/2
  Shift Arithmetic/1 -> Add3/2, Add2/2
  Logical Operator1/1 -> Switch1/2
  ANGLE/1 -> Add6/2, Add5/2

== system OFDM_Rx/OFDMRx/PhaseTracking_2/CordicRotate/Cell7 ==
  X_in_0 : Inport
  Y_in_0 : Inport  Port=2
  Ang_in_0 : Inport  Port=3
  ANGLE : Constant  Value=0.007812341060101  VectorParams1D=off  OutDataTypeStr=fixdt(1,23,20)  SampleTime=1/fs
  Add1 : Sum  Inputs=+-  OutDataTypeStr=fixdt(1,21,15)
  Add2 : Sum  OutDataTypeStr=fixdt(1,21,15)
  Add3 : Sum  Inputs=+-  OutDataTypeStr=fixdt(1,21,15)
  Add4 : Sum  OutDataTypeStr=fixdt(1,21,15)
  Add5 : Sum  OutDataTypeStr=fixdt(1,23,20)
  Add6 : Sum  Inputs=+-  OutDataTypeStr=fixdt(1,23,20)
  Compare To Constant : simulink/Logic and Bit Operations/Compare To Constant  relop=<  const=0  OutDataTypeStr=boolean
  Logical Operator1 : Logic  Operator=NOT  IconShape=distinctive  AllPortsSameDT=off  OutDataTypeStr=boolean
  Shift Arithmetic : ArithShift  BitShiftNumber=7
  Shift Arithmetic1 : ArithShift  BitShiftNumber=7
  Switch : Switch  Criteria=u2 ~= 0
  Switch1 : Switch  Criteria=u2 ~= 0
  Switch2 : Switch  Criteria=u2 ~= 0
  X_out_0 : Outport  VectorParamsAs1DForOutWhenUnconnected=off
  Y_out_0 : Outport  Port=2  VectorParamsAs1DForOutWhenUnconnected=off
  Ang_out_0 : Outport  Port=3  VectorParamsAs1DForOutWhenUnconnected=off
  wires:
  ANGLE/1 -> Add5/2, Add6/2
  Logical Operator1/1 -> Switch1/2
  Shift Arithmetic/1 -> Add2/2, Add3/2
  Shift Arithmetic1/1 -> Add4/2, Add1/2
  Compare To Constant/1 -> Switch2/2, Switch/2, Logical Operator1/1
  Ang_in_0/1 -> Compare To Constant/1, Add5/1, Add6/1
  Y_in_0/1 -> Add2/1, Add3/1, Shift Arithmetic1/1
  X_in_0/1 -> Add4/1, Add1/1, Shift Arithmetic/1
  Switch2/1 -> Ang_out_0/1
  Add5/1 -> Switch2/1
  Add6/1 -> Switch2/3
  Switch1/1 -> Y_out_0/1
  Switch/1 -> X_out_0/1
  Add2/1 -> Switch1/1
  Add3/1 -> Switch1/3
  Add1/1 -> Switch/3
  Add4/1 -> Switch/1

== system OFDM_Rx/OFDMRx/PhaseTracking_2/CordicRotate/Cell8 ==
  X_in_0 : Inport
  Y_in_0 : Inport  Port=2
  Ang_in_0 : Inport  Port=3
  ANGLE : Constant  Value=0.003906230131967  VectorParams1D=off  OutDataTypeStr=fixdt(1,23,20)  SampleTime=1/fs
  Add1 : Sum  Inputs=+-  OutDataTypeStr=fixdt(1,21,15)
  Add2 : Sum  OutDataTypeStr=fixdt(1,21,15)
  Add3 : Sum  Inputs=+-  OutDataTypeStr=fixdt(1,21,15)
  Add4 : Sum  OutDataTypeStr=fixdt(1,21,15)
  Add5 : Sum  OutDataTypeStr=fixdt(1,23,20)
  Add6 : Sum  Inputs=+-  OutDataTypeStr=fixdt(1,23,20)
  Compare To Constant : simulink/Logic and Bit Operations/Compare To Constant  relop=<  const=0  OutDataTypeStr=boolean
  Logical Operator1 : Logic  Operator=NOT  IconShape=distinctive  AllPortsSameDT=off  OutDataTypeStr=boolean
  Shift Arithmetic : ArithShift  BitShiftNumber=8
  Shift Arithmetic1 : ArithShift  BitShiftNumber=8
  Switch : Switch  Criteria=u2 ~= 0
  Switch1 : Switch  Criteria=u2 ~= 0
  Switch2 : Switch  Criteria=u2 ~= 0
  X_out_0 : Outport  VectorParamsAs1DForOutWhenUnconnected=off
  Y_out_0 : Outport  Port=2  VectorParamsAs1DForOutWhenUnconnected=off
  Ang_out_0 : Outport  Port=3  VectorParamsAs1DForOutWhenUnconnected=off
  wires:
  Add4/1 -> Switch/1
  Add1/1 -> Switch/3
  Add3/1 -> Switch1/3
  Add2/1 -> Switch1/1
  Switch/1 -> X_out_0/1
  Switch1/1 -> Y_out_0/1
  Add6/1 -> Switch2/3
  Add5/1 -> Switch2/1
  Switch2/1 -> Ang_out_0/1
  X_in_0/1 -> Shift Arithmetic/1, Add1/1, Add4/1
  Y_in_0/1 -> Shift Arithmetic1/1, Add3/1, Add2/1
  Ang_in_0/1 -> Add6/1, Add5/1, Compare To Constant/1
  Compare To Constant/1 -> Logical Operator1/1, Switch/2, Switch2/2
  Shift Arithmetic1/1 -> Add1/2, Add4/2
  Shift Arithmetic/1 -> Add3/2, Add2/2
  Logical Operator1/1 -> Switch1/2
  ANGLE/1 -> Add6/2, Add5/2

== system OFDM_Rx/OFDMRx/PhaseTracking_2/CordicRotate/Cell9 ==
  X_in_0 : Inport
  Y_in_0 : Inport  Port=2
  Ang_in_0 : Inport  Port=3
  ANGLE : Constant  Value=0.001953122516479  VectorParams1D=off  OutDataTypeStr=fixdt(1,23,20)  SampleTime=1/fs
  Add1 : Sum  Inputs=+-  OutDataTypeStr=fixdt(1,21,15)
  Add2 : Sum  OutDataTypeStr=fixdt(1,21,15)
  Add3 : Sum  Inputs=+-  OutDataTypeStr=fixdt(1,21,15)
  Add4 : Sum  OutDataTypeStr=fixdt(1,21,15)
  Add5 : Sum  OutDataTypeStr=fixdt(1,23,20)
  Add6 : Sum  Inputs=+-  OutDataTypeStr=fixdt(1,23,20)
  Compare To Constant : simulink/Logic and Bit Operations/Compare To Constant  relop=<  const=0  OutDataTypeStr=boolean
  Logical Operator1 : Logic  Operator=NOT  IconShape=distinctive  AllPortsSameDT=off  OutDataTypeStr=boolean
  Shift Arithmetic : ArithShift  BitShiftNumber=9
  Shift Arithmetic1 : ArithShift  BitShiftNumber=9
  Switch : Switch  Criteria=u2 ~= 0
  Switch1 : Switch  Criteria=u2 ~= 0
  Switch2 : Switch  Criteria=u2 ~= 0
  X_out_0 : Outport  VectorParamsAs1DForOutWhenUnconnected=off
  Y_out_0 : Outport  Port=2  VectorParamsAs1DForOutWhenUnconnected=off
  Ang_out_0 : Outport  Port=3  VectorParamsAs1DForOutWhenUnconnected=off
  wires:
  ANGLE/1 -> Add5/2, Add6/2
  Logical Operator1/1 -> Switch1/2
  Shift Arithmetic/1 -> Add2/2, Add3/2
  Shift Arithmetic1/1 -> Add4/2, Add1/2
  Compare To Constant/1 -> Switch2/2, Switch/2, Logical Operator1/1
  Ang_in_0/1 -> Compare To Constant/1, Add5/1, Add6/1
  Y_in_0/1 -> Add2/1, Add3/1, Shift Arithmetic1/1
  X_in_0/1 -> Add4/1, Add1/1, Shift Arithmetic/1
  Switch2/1 -> Ang_out_0/1
  Add5/1 -> Switch2/1
  Add6/1 -> Switch2/3
  Switch1/1 -> Y_out_0/1
  Switch/1 -> X_out_0/1
  Add2/1 -> Switch1/1
  Add3/1 -> Switch1/3
  Add1/1 -> Switch/3
  Add4/1 -> Switch/1

== system OFDM_Rx/OFDMRx/PhaseTracking_2/CordicRotate/GAIN_CORR ==
  XIN : Inport
  Constant : Constant  Value=0.607253321089875  OutDataTypeStr=fixdt(1,18,17)  SampleTime=1/fs
  Product : Product  OutDataTypeStr=fixdt(1,16,14)
  XOUT : Outport  VectorParamsAs1DForOutWhenUnconnected=off
  wires:
  Product/1 -> XOUT/1
  XIN/1 -> Product/2
  Constant/1 -> Product/1

== system OFDM_Rx/OFDMRx/PhaseTracking_2/CordicRotate/GAIN_CORR1 ==
  YIN : Inport
  Constant : Constant  Value=0.607253321089875  OutDataTypeStr=fixdt(1,18,17)  SampleTime=1/fs
  Product : Product  OutDataTypeStr=fixdt(1,16,14)
  YOUT : Outport  VectorParamsAs1DForOutWhenUnconnected=off
  wires:
  Product/1 -> YOUT/1
  Constant/1 -> Product/1
  YIN/1 -> Product/2

== system OFDM_Rx/OFDMRx/PhaseTracking_2/CordicRotate/QCORR ==
  X_in : Inport
  Y_in : Inport  Port=2
  Ctrl_in : Inport  Port=3
  QUAD_MAP1 : MATLAB Function  TreatAsAtomicUnit=on
  X_out : Outport  VectorParamsAs1DForOutWhenUnconnected=off
  Y_out : Outport  Port=2  VectorParamsAs1DForOutWhenUnconnected=off
  wires:
  Ctrl_in/1 -> QUAD_MAP1/3(ctrl)
  Y_in/1 -> QUAD_MAP1/2(yin)
  X_in/1 -> QUAD_MAP1/1(xin)
  QUAD_MAP1/1(xout) -> X_out/1
  QUAD_MAP1/2(yout) -> Y_out/1

== system OFDM_Rx/OFDMRx/PhaseTracking_2/CordicRotate/QUAD_MAP ==
  Xin : Inport
  Yin : Inport  Port=2
  ANG_IN : Inport  Port=3
  QUAD_DETERM1 : MATLAB Function  TreatAsAtomicUnit=on
  Xout : Outport  VectorParamsAs1DForOutWhenUnconnected=off
  Yout : Outport  Port=2  VectorParamsAs1DForOutWhenUnconnected=off
  ANG_OUT : Outport  Port=3  VectorParamsAs1DForOutWhenUnconnected=off
  QUAD_CTRL_OUT : Outport  Port=4  VectorParamsAs1DForOutWhenUnconnected=off
  wires:
  ANG_IN/1 -> QUAD_DETERM1/1(ang_in)
  QUAD_DETERM1/1(ang_out) -> ANG_OUT/1
  Xin/1 -> Xout/1
  Yin/1 -> Yout/1
  QUAD_DETERM1/2(QUAD) -> QUAD_CTRL_OUT/1

== system OFDM_Rx/OFDMRx/PhaseTracking_2/PhaseEst/CIC_MA ==
  In1 : Inport
  Add : Sum  Inputs=-+  AccumDataTypeStr=fixdt(1,23,15)
  Add1 : Sum  AccumDataTypeStr=fixdt(1,23,15)
  Delay1 : Delay  DelayLength=4
  Delay2 : Delay  DelayLength=1
  Out1 : Outport  VectorParamsAs1DForOutWhenUnconnected=off
  wires:
  Add1/1 -> Delay2/1
  Add/1 -> Add1/2
  Delay1/1 -> Add/1
  In1/1 -> Add/2, Delay1/1
  Delay2/1 -> Add1/1, Out1/1

== system OFDM_Rx/OFDMRx/PhaseTracking_2/PilotCtrlGen/CtrlSigGen ==
  valid : Inport
  sampleCount : Inport  Port=2
  Compare To Constant1 : simulink/Logic and Bit Operations/Compare To Constant  relop===  const=3  OutDataTypeStr=boolean
  Compare To Constant4 : simulink/Logic and Bit Operations/Compare To Constant  relop=>=  const=4  OutDataTypeStr=boolean
  Compare To Constant5 : simulink/Logic and Bit Operations/Compare To Constant  relop=<=  const=51  OutDataTypeStr=boolean
  Logical Operator2 : Logic  IconShape=distinctive  AllPortsSameDT=off  OutDataTypeStr=boolean
  Logical Operator4 : Logic  IconShape=distinctive  AllPortsSameDT=off  OutDataTypeStr=boolean
  Logical Operator5 : Logic  IconShape=distinctive  AllPortsSameDT=off  OutDataTypeStr=boolean
  dataValid : Outport
  pilotEnd : Outport  Port=2
  wires:
  valid/1 -> Logical Operator5/1, Logical Operator4/1
  sampleCount/1 -> Compare To Constant4/1, Compare To Constant5/1, Compare To Constant1/1
  Logical Operator4/1 -> dataValid/1
  Logical Operator2/1 -> Logical Operator4/2
  Compare To Constant1/1 -> Logical Operator5/2
  Compare To Constant4/1 -> Logical Operator2/1
  Logical Operator5/1 -> pilotEnd/1
  Compare To Constant5/1 -> Logical Operator2/2

== system OFDM_Rx/OFDMRx/PhaseTracking_2/PilotCtrlGen/SampleCounter ==
  Valid_In : Inport
  Delay : Delay  DelayLength=1
  Logical Operator : Logic  Operator=NOT  IconShape=distinctive  AllPortsSameDT=off  OutDataTypeStr=boolean
  SAMPLE_COUNTER : hdlsllib/Sources/HDL Counter  CountType=Count limited  CountInit=0  CountStep=1  CountMax=51  CountFromType=Initial value  CountFrom=0  CountResetPort=on  CountLoadPort=off  CountEnbPort=on  CountDirPort=off  CountDataType=Unsigned  CountWordLen=6  CountFracLen=0  CountSampTime=1
  Sample_Cnt : Outport  VectorParamsAs1DForOutWhenUnconnected=off
  wires:
  Delay/1 -> Sample_Cnt/1
  Logical Operator/1 -> SAMPLE_COUNTER/1
  Valid_In/1 -> SAMPLE_COUNTER/2, Logical Operator/1
  SAMPLE_COUNTER/1 -> Delay/1

== system OFDM_Rx/OFDMRx/PhaseTracking_2/PilotCtrlGen/SymbolCounter ==
  ValidIn : Inport
  Delay : Delay  DelayLength=1
  HDL Counter : hdlsllib/Sources/HDL Counter  CountType=Count limited  CountInit=0  CountStep=1  CountMax=126  CountFromType=Initial value  CountFrom=0  CountResetPort=off  CountLoadPort=off  CountEnbPort=on  CountDirPort=off  CountDataType=Unsigned  CountWordLen=7  CountFracLen=0  CountSampTime=1
  Relational Operator : RelationalOperator  Operator=<  OutDataTypeStr=boolean  RndMeth=Nearest
  Symbl_cnt : Outport  VectorParamsAs1DForOutWhenUnconnected=off
  wires:
  Relational Operator/1 -> HDL Counter/1
  HDL Counter/1 -> Symbl_cnt/1
  Delay/1 -> Relational Operator/2
  ValidIn/1 -> Delay/1, Relational Operator/1

== system OFDM_Rx/OFDMRx/PhaseTracking_2/PilotCtrlGen/pilotGen ==
  symbCount : Inport
  sampleCount : Inport  Port=2
  valid : Inport  Port=3
  Compare To Constant : simulink/Logic and Bit Operations/Compare To Constant  relop=>  const=0  OutDataTypeStr=boolean
  Compare To Constant2 : simulink/Logic and Bit Operations/Compare To Constant  relop=>=  const=0  OutDataTypeStr=boolean
  Compare To Constant3 : simulink/Logic and Bit Operations/Compare To Constant  relop=<  const=4  OutDataTypeStr=boolean
  Constant : Constant  Value=0  OutDataTypeStr=fixdt(1,2,0)  SampleTime=1/fs
  HDL Counter1 : hdlsllib/Sources/HDL Counter  CountType=Count limited  CountInit=0  CountStep=1  CountMax=3  CountFromType=Initial value  CountFrom=0  CountResetPort=off  CountLoadPort=off  CountEnbPort=on  CountDirPort=off  CountDataType=Unsigned  CountWordLen=2  CountFracLen=0  CountSampTime=1
  Logical Operator1 : Logic  IconShape=distinctive  AllPortsSameDT=off  OutDataTypeStr=boolean
  Logical Operator3 : Logic  IconShape=distinctive  AllPortsSameDT=off  OutDataTypeStr=boolean
  PilotValue_LUT1 : Lookup_n-D  NumberOfTableDimensions=1  LookupTableObject=''  BreakpointsForDimension1=[0:3]  BreakpointsForDimension1FirstPoint=10  BreakpointsForDimension2FirstPoint=10  BreakpointsForDimension1Spacing=12  BreakpointsForDimension2Spacing=12  IndexSearchMethod=Evenly spaced points  Table=[1 1 1 -1]  TableDataTypeStr=fixdt(1,2,0)  InterpMethod=Flat  DiagnosticForOutOfRangeInput=Error  InternalRulePriority=Speed  OutDataTypeStr=fixdt(1,2,0)  RndMeth=Simplest  InputSameDT=on
  Polarity_LUT1 : Lookup_n-D  NumberOfTableDimensions=1  LookupTableObject=''  BreakpointsForDimension1=[0:126]  BreakpointsForDimension1FirstPoint=10  BreakpointsForDimension2FirstPoint=10  BreakpointsForDimension1Spacing=12  BreakpointsForDimension2Spacing=12  IndexSearchMethod=Evenly spaced points  Table=pilot  TableDataTypeStr=fixdt(1,2,0)  InterpMethod=Flat  DiagnosticForOutOfRangeInput=Error  InternalRulePriority=Speed  OutDataTypeStr=fixdt(1,2,0)  RndMeth=Simplest  InputSameDT=on
  Switch : Switch  Criteria=u2 ~= 0
  Switch1 : Switch  Criteria=u2 ~= 0
  ToComplex1 : Subsystem
  Unary Minus : UnaryMinus
  pilOut : Outport
  wires:
  Logical Operator3/1 -> HDL Counter1/1, Switch1/2
  valid/1 -> Logical Operator3/1
  Compare To Constant3/1 -> Logical Operator1/2
  Compare To Constant2/1 -> Logical Operator1/1
  Logical Operator1/1 -> Logical Operator3/2
  sampleCount/1 -> Compare To Constant3/1, Compare To Constant2/1
  symbCount/1 -> Polarity_LUT1/1
  Constant/1 -> Switch1/3
  Switch1/1 -> Switch/1, Unary Minus/1
  ToComplex1/1(Out1) -> pilOut/1
  Compare To Constant/1 -> Switch/2
  Unary Minus/1 -> Switch/3
  Switch/1 -> ToComplex1/1(In1)
  PilotValue_LUT1/1 -> Switch1/1
  Polarity_LUT1/1 -> Compare To Constant/1
  HDL Counter1/1 -> PilotValue_LUT1/1

== system OFDM_Rx/OFDMRx/Synchronisation/CoarseFreqCorr/RsingEdge ==
  In1 : Inport
  Delay : Delay  DelayLength=1
  Relational Operator : RelationalOperator  Operator=>  OutDataTypeStr=boolean  RndMeth=Nearest
  Out1 : Outport  VectorParamsAs1DForOutWhenUnconnected=off
  wires:
  In1/1 -> Relational Operator/1, Delay/1
  Delay/1 -> Relational Operator/2
  Relational Operator/1 -> Out1/1

== system OFDM_Rx/OFDMRx/Synchronisation/ControlSigGen/PreambleValidGen ==
  ValidIn : Inport
  Compare To Constant : simulink/Logic and Bit Operations/Compare To Constant  relop===  const=128  OutDataTypeStr=boolean
  HDL Counter : hdlsllib/Sources/HDL Counter  CountType=Count limited  CountInit=0  CountStep=1  CountMax=128  CountFromType=Initial value  CountFrom=0  CountResetPort=on  CountLoadPort=off  CountEnbPort=on  CountDirPort=off  CountDataType=Unsigned  CountWordLen=8  CountFracLen=0  CountSampTime=1
  NOT : Logic  Operator=NOT  IconShape=distinctive  AllPortsSameDT=off  OutDataTypeStr=boolean
  RisingEdge : Subsystem
  Unit Delay Enabled Resettable Synchronous : hdlsllib/Discrete/Unit Delay Enabled Resettable Synchronous  InitialCondition=0.0  SampleTime=-1
      settings: SourceProductBaseCode=SL
  y : Outport
  wires:
  HDL Counter/1 -> Compare To Constant/1
  RisingEdge/1(Out1) -> Unit Delay Enabled Resettable Synchronous/2
  NOT/1 -> HDL Counter/1
  Compare To Constant/1 -> Unit Delay Enabled Resettable Synchronous/3
  ValidIn/1 -> RisingEdge/1(ValidIn), NOT/1, HDL Counter/2, Unit Delay Enabled Resettable Synchronous/1
  Unit Delay Enabled Resettable Synchronous/1 -> y/1

== system OFDM_Rx/OFDMRx/Synchronisation/ControlSigGen/dataValidGen ==
  enb : Inport
  enb1 : Inport  Port=2
  AND : Logic  IconShape=distinctive  AllPortsSameDT=off  OutDataTypeStr=boolean
  Compare To Constant : simulink/Logic and Bit Operations/Compare To Constant  relop=>  const=15  OutDataTypeStr=boolean
  Delay : Delay  DelayLength=1
  HDL Counter : hdlsllib/Sources/HDL Counter  CountType=Count limited  CountInit=0  CountStep=1  CountMax=79  CountFromType=Initial value  CountFrom=0  CountResetPort=on  CountLoadPort=off  CountEnbPort=on  CountDirPort=off  CountDataType=Unsigned  CountWordLen=7  CountFracLen=0  CountSampTime=1
  NOT : Logic  Operator=NOT  IconShape=distinctive  AllPortsSameDT=off  OutDataTypeStr=boolean
  NOT1 : Logic  Operator=NOT  IconShape=distinctive  AllPortsSameDT=off  OutDataTypeStr=boolean
  y : Outport
  wires:
  enb/1 -> NOT1/1
  enb1/1 -> Delay/1
  Delay/1 -> AND/2
  AND/1 -> HDL Counter/2, NOT/1
  NOT1/1 -> AND/1
  Compare To Constant/1 -> y/1
  NOT/1 -> HDL Counter/1
  HDL Counter/1 -> Compare To Constant/1

== system OFDM_Rx/OFDMRx/Synchronisation/FrameDetect/RsingEdge ==
  In1 : Inport
  Constant : Constant  OutDataTypeStr=boolean  SampleTime=1/fs
  Constant1 : Constant  Value=0  OutDataTypeStr=boolean  SampleTime=1/fs
  Delay : Delay  DelayLength=1
  Relational Operator : RelationalOperator  Operator=>  OutDataTypeStr=boolean  RndMeth=Nearest
  Unit Delay Enabled Resettable Synchronous : hdlsllib/Discrete/Unit Delay Enabled Resettable Synchronous  InitialCondition=0.0  SampleTime=-1
      settings: SourceProductBaseCode=SL
  Out1 : Outport  VectorParamsAs1DForOutWhenUnconnected=off
  wires:
  Constant1/1 -> Unit Delay Enabled Resettable Synchronous/3
  Constant/1 -> Unit Delay Enabled Resettable Synchronous/1
  Unit Delay Enabled Resettable Synchronous/1 -> Out1/1
  In1/1 -> Relational Operator/1, Delay/1
  Delay/1 -> Relational Operator/2
  Relational Operator/1 -> Unit Delay Enabled Resettable Synchronous/2

== system OFDM_Rx/OFDMRx/Synchronisation/SchmidlCoxMetric /Abs2 ==
  Abs2In : Inport
  Add : Sum  OutDataTypeStr=fixdt(0,25,23)
  Complex to Real-Imag : ComplexToRealImag
  Delay{1..4} (4 alike) : Delay  DelayLength=1
  Delay5 : Delay
  Product : Product  OutDataTypeStr=fixdt(0,25,23)
  Product1 : Product  OutDataTypeStr=fixdt(0,25,23)
  Abs2Out : Outport  VectorParamsAs1DForOutWhenUnconnected=off
  wires:
  Abs2In/1 -> Complex to Real-Imag/1
  Complex to Real-Imag/1 -> Delay1/1
  Complex to Real-Imag/2 -> Delay2/1
  Product/1 -> Delay3/1
  Product1/1 -> Delay4/1
  Add/1 -> Delay5/1
  Delay1/1 -> Product/1, Product/2
  Delay2/1 -> Product1/2, Product1/1
  Delay3/1 -> Add/1
  Delay4/1 -> Add/2
  Delay5/1 -> Abs2Out/1

== system OFDM_Rx/OFDMRx/Synchronisation/SchmidlCoxMetric /AutoCorr ==
  AcorrIn : Inport
  Delay : Delay  DelayLength=16
  Delay{1..5} (5 alike) : Delay  DelayLength=1
  Math Function : Math  Operator=conj  SignedPower=on  RndMeth=Zero  SaturateOnIntegerOverflow=on
  Product : Product  OutDataTypeStr=fixdt(1,25,23)
  AcorrOut : Outport  VectorParamsAs1DForOutWhenUnconnected=off
  wires:
  AcorrIn/1 -> Delay1/1
  Math Function/1 -> Delay4/1
  Product/1 -> Delay5/1
  Delay/1 -> Math Function/1
  Delay1/1 -> Delay/1, Delay3/1
  Delay2/1 -> AcorrOut/1
  Delay3/1 -> Product/1
  Delay4/1 -> Product/2
  Delay5/1 -> Delay2/1

== system OFDM_Rx/OFDMRx/Synchronisation/SchmidlCoxMetric /CIC_ma ==
  note: The averaging window is set to 64 samples i.e.
      | 4x repetitions of the L-STF. Using a larger averaging
      | window improves the coarse CFO estimate. This
      | approach leaves 6x L-STF repetitions for AGC convergence.
  In1 : Inport
  Add : Sum  Inputs=-+  AccumDataTypeStr=fixdt(1,33,23)
  Add1 : Sum  AccumDataTypeStr=fixdt(1,33,23)
  Data Type Conversion : DataTypeConversion  OutDataTypeStr=fixdt(1,18,16)
  Delay1 : Delay  DelayLength=48
  Delay2 : Delay  DelayLength=1
  Delay3 : Delay  DelayLength=1
  Delay4 : Delay  DelayLength=1
  Out1 : Outport  VectorParamsAs1DForOutWhenUnconnected=off
  wires:
  Add/1 -> Add1/2
  Delay1/1 -> Add/1
  In1/1 -> Delay3/1
  Add1/1 -> Delay2/1
  Delay2/1 -> Delay4/1, Add1/1
  Delay3/1 -> Add/2, Delay1/1
  Delay4/1 -> Data Type Conversion/1
  Data Type Conversion/1 -> Out1/1

== system OFDM_Rx/OFDMRx/Synchronisation/SchmidlCoxMetric /CIC_ma1 ==
  In1 : Inport
  Add : Sum  Inputs=-+  AccumDataTypeStr=fixdt(1,33,23)
  Add1 : Sum  AccumDataTypeStr=fixdt(1,33,23)
  Data Type Conversion : DataTypeConversion  OutDataTypeStr=fixdt(1,18,15)
  Delay1 : Delay  DelayLength=48
  Delay2 : Delay  DelayLength=1
  Delay3 : Delay  DelayLength=1
  Delay4 : Delay  DelayLength=1
  Out1 : Outport  VectorParamsAs1DForOutWhenUnconnected=off
  wires:
  Delay2/1 -> Add1/1, Delay4/1
  Add1/1 -> Delay2/1
  In1/1 -> Delay3/1
  Delay1/1 -> Add/1
  Add/1 -> Add1/2
  Delay3/1 -> Delay1/1, Add/2
  Delay4/1 -> Data Type Conversion/1
  Data Type Conversion/1 -> Out1/1
